simulink model "pendule_simple"  (R2015a)
settings: Solver=ode3  StartTime=0.0  StopTime=10.0  FixedStep=0.01  RelTol=1e-3
undefined symbols (not defined in the file): l
libraries: simulink x1
settings Model: Creator=fschalle  LastModifiedBy=root

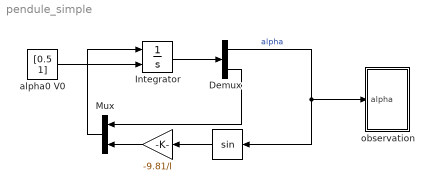
== system pendule_simple ==
  "   " : Trigonometry
  " " : Gain  Gain=-9.81/l
  Demux : Demux  Outputs=2
  Integrator : Integrator  InitialConditionSource=external
  Mux : Mux  Inputs=2
  alpha0 V0 : Constant  Value=[0.5 1]
  observation : Subsystem
  wires:
  alpha0 V0/1 -> Integrator/2
  Integrator/1 -> Demux/1
  " "/1 -> Mux/2
  Mux/1 -> Integrator/1
  "   "/1 -> " "/1
  Demux/1 -> "   "/1, observation/1(alpha)  "alpha"
  Demux/2 -> Mux/1

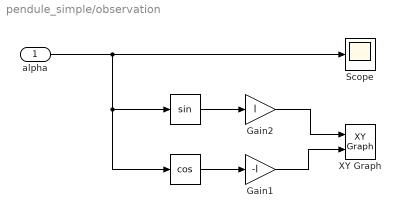
== system pendule_simple/observation ==
  alpha : Inport
  " " : Trigonometry
  "  " : Trigonometry  Operator=cos
  Gain1 : Gain  Gain=-l
  Gain2 : Gain  Gain=l
  Scope : Scope
      settings: YMin=-0.75  YMax=0.75
  XY Graph : simulink/Sinks/XY Graph  xmin=-1  xmax=1  ymin=-1  ymax=1  st=-1
  wires:
  alpha/1 -> "  "/1, " "/1, Scope/1
  Gain1/1 -> XY Graph/2
  " "/1 -> Gain2/1
  "  "/1 -> Gain1/1
  Gain2/1 -> XY Graph/1
